simulink model "sl_ztorque"  (R2019b)
settings: Solver=ode45  StartTime=0.0  StopTime=200  RelTol=1e-3  EnableMultiTasking=on
libraries: roblocks x4
settings Model: ExtModeTrigMode=oneshot  ExtModeArmWhenConnect=off  Creator=pic  LastModifiedBy=Karl
settings DataIOCC: SaveFormat=Array  SignalLoggingSaveFormat=ModelDataLogs  SignalLogging=off
settings OptimizationCC: BlockReduction=off  BooleanDataType=off  ExpressionDepthLimit=2147483647  InitFltsAndDblsToZero=on  LifeSpan=inf
settings DebuggingCC: SaveWithParameterizedLinksMsg=none  UnderspecifiedInitializationDetection=Classic  MergeDetectMultiDrivingBlocksExec=none  SignalResolutionControl=TryResolveAllWithWarning  MultiTaskDSMMsg=warning  MultiTaskCondExecSysMsg=none  FcnCallInpInsideContextMsg=warning  AllowSymbolicDim=off  StateNameClashWarn=warning  SFUnexpectedBacktrackingDiag=warning  SFNoUnconditionalDefaultTransitionDiag=warning  SFExecutionAtInitializationDiag=none  ArithmeticOperatorsInVariantConditions=warning
settings HardwareCC: ProdBitPerPointer=32  ProdBitPerSizeT=32  ProdBitPerPtrDiffT=32  ProdLargestAtomicFloat=None  ProdIntDivRoundTo=Undefined  ProdEndianess=Unspecified  ProdWordSize=32  ProdHWDeviceType=32-bit Generic  TargetUnknown=on
settings ModelReferenceCC: PropagateSignalLabelsOutOfModel=off
settings SFSimCC: SimUseLocalCustomCode=off  CustomCodeUndefinedFunction=UseInterfaceOnly
settings RTWCC: RTWUseLocalCustomCode=off
settings CodeAppCC: StateflowObjectComments=on
settings GRTTargetCC: TargetLangStandard=C89/C90 (ANSI)  ModelReferenceCompliant=off  ParMdlRefBuildCompliant=off  CompOptLevelCompliant=off  GeneratePreprocessorConditionals=Disable all  CombineOutputUpdateFcns=off  MatFileLogging=off  GRTInterface=on
settings ConfigComp: CovMetricSettings=dw  CovHtmlReporting=on  CovSaveCumulativeToWorkspaceVar=on  CovSaveSingleToWorkspaceVar=on  CovExternalEMLEnable=off  CovSFcnEnable=off

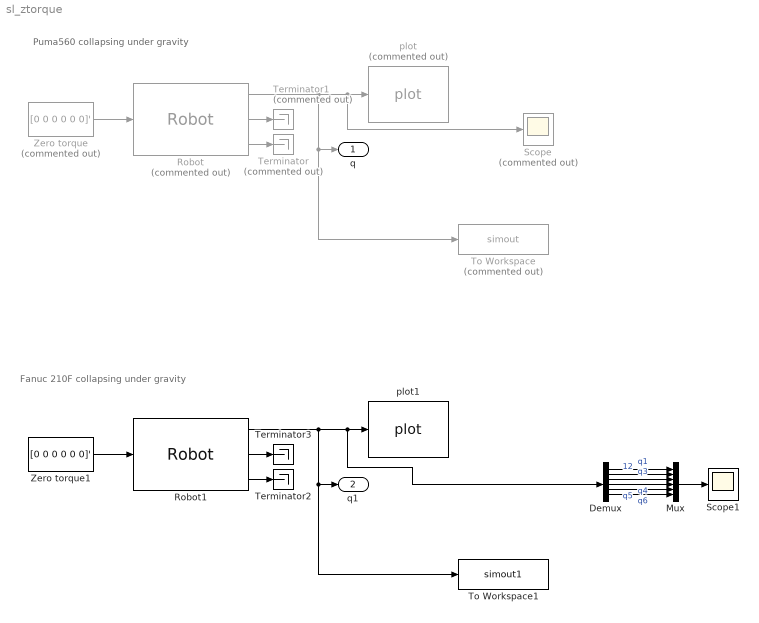
== system sl_ztorque ==
  note: Puma560 collapsing under gravity
  note: Fanuc 210F collapsing under gravity
  Demux : Demux  Outputs=6
  Mux : Mux  Inputs=6
  Robot : roblocks/Arm/Robot  Commented=on  robot=p560.nofriction  q0=[0 0 0 0 0 0]
  Robot1 : roblocks/Arm/Robot  robot=R.nofriction  q0=[0 0 0 0 0 0]
  Scope : Scope  Commented=on
  Scope1 : Scope
  Terminator : Terminator  Commented=on
  Terminator1 : Terminator  Commented=on
  Terminator2 : Terminator
  Terminator3 : Terminator
  To Workspace : ToWorkspace  Commented=on  VariableName=simout  SaveFormat=Timeseries  SampleTime=-1
  To Workspace1 : ToWorkspace  VariableName=simout1  SaveFormat=Timeseries  SampleTime=-1
  Zero torque : Constant  Commented=on  Value=[0 0 0 0 0 0]'
  Zero torque1 : Constant  Value=[0 0 0 0 0 0]'
  plot : roblocks/Arm/plot  Commented=on  robot=p560  fps=25  holdplot=on
  plot1 : roblocks/Arm/plot  robot=R  fps=25  holdplot=on
  q : Outport
  q1 : Outport  Port=2
  wires:
  Zero torque/1 -> Robot/1
  Robot/1 -> Scope/1, plot/1, To Workspace/1, q/1
  Robot/3 -> Terminator/1
  Robot/2 -> Terminator1/1
  Zero torque1/1 -> Robot1/1
  Robot1/1 -> Demux/1, plot1/1, To Workspace1/1, q1/1
  Robot1/3 -> Terminator2/1
  Robot1/2 -> Terminator3/1
  Demux/1 -> Mux/1  "q1"
  Demux/2 -> Mux/2  "12"
  Demux/3 -> Mux/3  "q3"
  Demux/4 -> Mux/4  "q4"
  Demux/5 -> Mux/5  "q5"
  Demux/6 -> Mux/6  "q6"
  Mux/1 -> Scope1/1
